simulink model "kevin_simulation1d"  (R2018b)
settings: Solver=VariableStepAuto  StartTime=0.0  StopTime=180  RelTol=1e-3
values from neighbouring files (symbols this model uses):
  a_phi_1 = 2.831    [kevin_d_course_manouvers.m]
  a_phi_2 = -0.629    [kevin_d_course_manouvers.m]
  d = 1.5    [kevin_d_course_manouvers.m]
  g = 9.81    [kevin_d_course_manouvers.m]
  kd_phi = 1.979    [kevin_d_course_manouvers.m]
  ki_chi = 0.6549    [kevin_d_course_manouvers.m]
  ki_phi = 0    [kevin_d_course_manouvers.m]
  kp_chi = 3.284    [kevin_d_course_manouvers.m]
  kp_phi = -2    [kevin_d_course_manouvers.m]
  vg = 161.111    [kevin_d_course_manouvers.m]
libraries: simulink x1
settings Model: Creator=Kevin K. Kaldvansvik  LastModifiedBy=dino
settings SFSimCC: SimUseLocalCustomCode=off
settings RTWCC: RTWUseLocalCustomCode=off
settings CodeAppCC: StateflowObjectComments=on

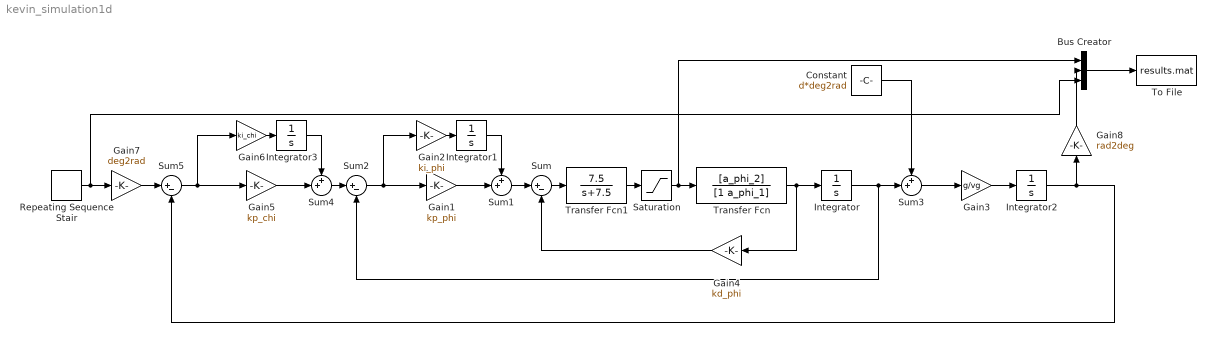
== system kevin_simulation1d ==
  Bus Creator : BusCreator  Inputs=3
  Constant : Constant  Value=d*deg2rad
  Gain1 : Gain  Gain=kp_phi
  Gain2 : Gain  Gain=ki_phi
  Gain3 : Gain  Gain=g/vg
  Gain4 : Gain  Gain=kd_phi
  Gain5 : Gain  Gain=kp_chi
  Gain6 : Gain  Gain=ki_chi
  Gain7 : Gain  Gain=deg2rad
  Gain8 : Gain  Gain=rad2deg
  Integrator{,1..3} (4 alike) : Integrator
  Repeating Sequence Stair : simulink/Sources/Repeating Sequence Stair  OutValues=[10 0 -10].'  tsamp=60  OutMin=[]  OutMax=[]  OutDataTypeStr=double  OutputDataTypeScalingMode=double  OutDataType=fixdt(0,8)  ConRadixGroup=Best Precision: Vector-wise  OutScaling=2^-12
  Saturation : Saturate  UpperLimit=30*deg2rad  LowerLimit=-30*deg2rad
  Sum : Sum  Inputs=|+-
  Sum1 : Sum  Inputs=++|
  Sum2 : Sum  Inputs=|+-
  Sum3 : Sum  Inputs=++|
  Sum4 : Sum  Inputs=++|
  Sum5 : Sum  Inputs=|+-
  To File : ToFile  Filename=results.mat
  Transfer Fcn : TransferFcn  Numerator=[a_phi_2]  Denominator=[1 a_phi_1]
  Transfer Fcn1 : TransferFcn  Numerator=[7.5]  Denominator=[1 7.5]
  wires:
  Transfer Fcn/1 -> Gain4/1, Integrator/1
  Sum1/1 -> Sum/1
  Gain1/1 -> Sum1/2
  Gain2/1 -> Integrator1/1
  Integrator1/1 -> Sum1/1
  Sum2/1 -> Gain2/1, Gain1/1
  Sum4/1 -> Sum2/1
  Integrator/1 -> Sum2/2, Sum3/2
  Constant/1 -> Sum3/1
  Sum3/1 -> Gain3/1
  Gain3/1 -> Integrator2/1
  Integrator2/1 -> Gain8/1, Sum5/2
  Gain4/1 -> Sum/2
  Gain5/1 -> Sum4/2
  Gain6/1 -> Integrator3/1
  Integrator3/1 -> Sum4/1
  Sum5/1 -> Gain6/1, Gain5/1
  Bus Creator/1 -> To File/1
  Sum/1 -> Transfer Fcn1/1
  Transfer Fcn1/1 -> Saturation/1
  Saturation/1 -> Bus Creator/1, Transfer Fcn/1
  Repeating Sequence Stair/1 -> Gain7/1, Bus Creator/3
  Gain7/1 -> Sum5/1
  Gain8/1 -> Bus Creator/2
